simulink model "Lab3simuModels"  (R2024b)
settings: Solver=VariableStepAuto  StartTime=0.0  StopTime=10.0  RelTol=1e-3
libraries: commanapbnd3 x1
settings Model: Creator=cloud  LastModifiedBy=cloud

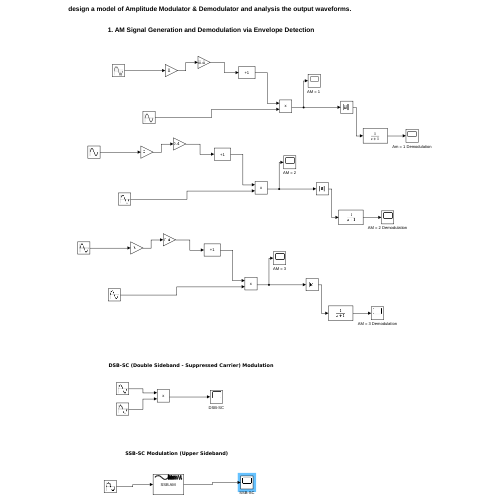
[thumbnail: Simulink's stored preview of the top-level diagram]
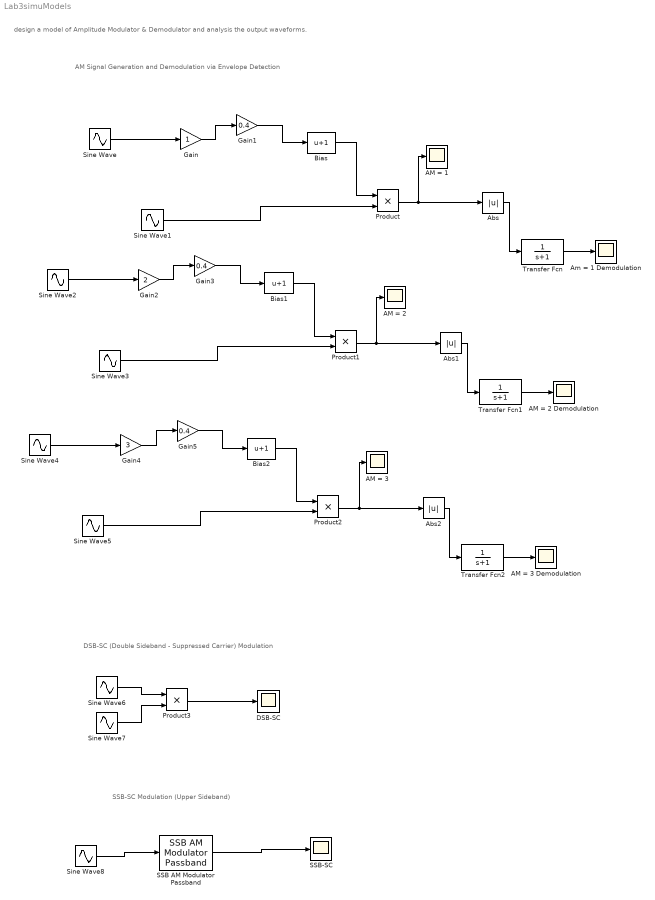
== system Lab3simuModels ==
  note: SSB-SC Modulation (Upper Sideband)
  note: DSB-SC (Double Sideband - Suppressed Carrier) Modulation
  note: AM Signal Generation and Demodulation via Envelope Detection
  note: design a model of Amplitude Modulator & Demodulator and analysis the output waveforms.
  "AM = 1 " : Scope
  AM = 2 : Scope
  AM = 2 Demodulation : Scope
  AM = 3 : Scope
  AM = 3 Demodulation : Scope
  Abs : Abs  SaturateOnIntegerOverflow=off
  Abs1 : Abs  SaturateOnIntegerOverflow=off
  Abs2 : Abs  SaturateOnIntegerOverflow=off
  Am = 1 Demodulation : Scope
  Bias : Bias  Bias=1  SaturateOnIntegerOverflow=off
  Bias1 : Bias  Bias=1  SaturateOnIntegerOverflow=off
  Bias2 : Bias  Bias=1  SaturateOnIntegerOverflow=off
  DSB-SC : Scope
  Gain : Gain
  Gain1 : Gain  Gain=0.4
  Gain2 : Gain  Gain=2
  Gain3 : Gain  Gain=0.4
  Gain4 : Gain  Gain=3
  Gain5 : Gain  Gain=0.4
  Product{,1..3} (4 alike) : Product
  SSB AM Modulator Passband : commanapbnd3/SSB AM Modulator Passband  Fc=100  Ph=0  Sd=Upper  Ho=100
  SSB-SC : Scope
  Sine Wave : Sin  Frequency=10  SampleTime=0
  Sine Wave{1,3,5,7} (4 alike) : Sin  Frequency=100  SampleTime=0
  Sine Wave2 : Sin  Frequency=10  SampleTime=0
  Sine Wave4 : Sin  Frequency=10  SampleTime=0
  Sine Wave6 : Sin  Amplitude=2  Frequency=10  SampleTime=0
  Sine Wave8 : Sin  Frequency=10  SampleTime=0.0001
  Transfer Fcn : TransferFcn  Denominator=[1 1]
  Transfer Fcn1 : TransferFcn  Denominator=[1 1]
  Transfer Fcn2 : TransferFcn  Denominator=[1 1]
  wires:
  Gain/1 -> Gain1/1
  Gain1/1 -> Bias/1
  Bias/1 -> Product/1
  Sine Wave1/1 -> Product/2
  Sine Wave/1 -> Gain/1
  Product/1 -> "AM = 1 "/1, Abs/1
  Abs/1 -> Transfer Fcn/1
  Transfer Fcn/1 -> Am = 1 Demodulation/1
  Abs1/1 -> Transfer Fcn1/1
  Sine Wave3/1 -> Product1/2
  Gain2/1 -> Gain3/1
  Product1/1 -> AM = 2/1, Abs1/1
  Sine Wave2/1 -> Gain2/1
  Transfer Fcn1/1 -> AM = 2 Demodulation/1
  Bias1/1 -> Product1/1
  Gain3/1 -> Bias1/1
  Abs2/1 -> Transfer Fcn2/1
  Sine Wave5/1 -> Product2/2
  Gain4/1 -> Gain5/1
  Product2/1 -> AM = 3/1, Abs2/1
  Sine Wave4/1 -> Gain4/1
  Transfer Fcn2/1 -> AM = 3 Demodulation/1
  Bias2/1 -> Product2/1
  Gain5/1 -> Bias2/1
  Sine Wave6/1 -> Product3/1
  Sine Wave7/1 -> Product3/2
  Product3/1 -> DSB-SC/1
  Sine Wave8/1 -> SSB AM Modulator Passband/1
  SSB AM Modulator Passband/1 -> SSB-SC/1
